simulink model "doc_evm"  (R2014a)
settings: Solver=FixedStepDiscrete  StartTime=0.0  StopTime=(paramEVM.numBursts)*paramEVM.burstLen2*paramEVM.Tnormal  FixedStep=paramEVM.Tnormal  MaxStep=paramEVM.Tnormal  RelTol=1e-3
PreLoadFcn:
  |  paramEVM = doc_evm_init;
undefined symbols (not defined in the file or in its folder): commblksprivate, dfilt, Info
libraries: commrflib2 x3, dsparch4 x2, commutil2 x1, commdigbbndpm3 x1, dspstat3 x1, commrandsrc2 x1, dspsigops x1
CloseFcn:
  | clear paramEVM;
settings Model: Creator=The MathWorks Inc.
settings DataIOCC: SignalLoggingSaveFormat=ModelDataLogs
settings OptimizationCC: ExpressionDepthLimit=2147483647
settings DebuggingCC: UnderspecifiedInitializationDetection=Classic  FcnCallInpInsideContextMsg=UseLocalSettings  StateNameClashWarn=warning  StrictBusMsg=Warning
settings SFSimCC: SimParseCustomCode=off
settings GRTTargetCC: CombineOutputUpdateFcns=off  GRTInterface=on

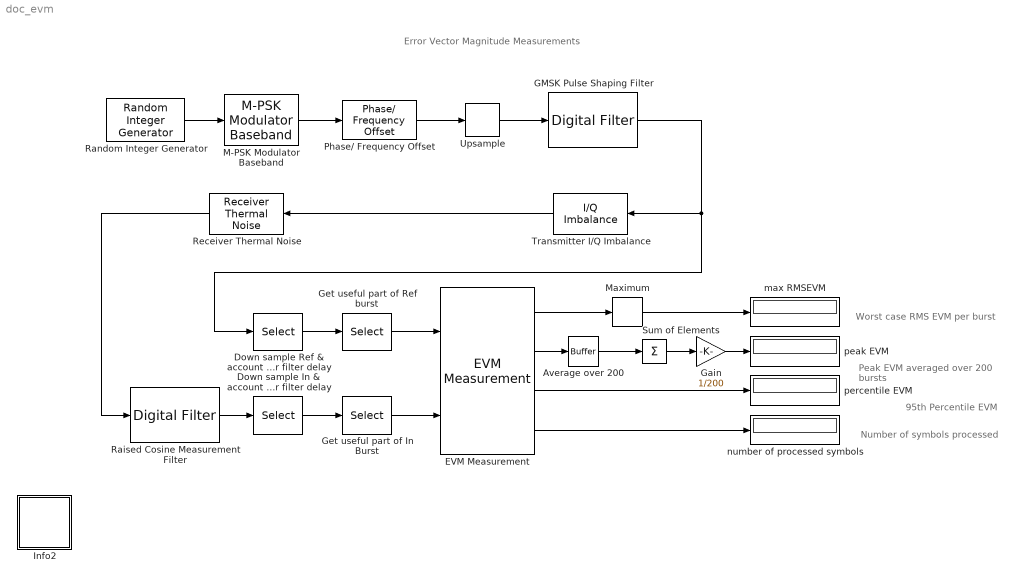
== system doc_evm ==
  note: Error Vector Magnitude Measurements
  note: Worst case
      | RMS EVM per burst
  note: Peak EVM
      | averaged over 200 bursts
  note: 95th Percentile EVM
  note: Number of
      | symbols processed
  Average over 200 : Buffer  N=200  TreatMby1Signals=One channel
  Down sample In & account for filter delay : Selector  NumberOfDimensions=2  InputPortWidth=3  IndexOptions=Index vector (dialog),Select all  Indices=[paramEVM.rcvSigDelay+1:paramEVM.Nsamp:paramEVM.burstLen2*paramEVM.Nsamp],1  OutputSizes=1,1
  Down sample Ref & account for filter delay : Selector  NumberOfDimensions=2  InputPortWidth=3  IndexOptions=Index vector (dialog),Select all  Indices=[paramEVM.refSigDelay+1:paramEVM.Nsamp:paramEVM.burstLen2*paramEVM.Nsamp],1  OutputSizes=1,1
  EVM Measurement : commutil2/EVM Measurement  normMethod=Average reference signal power  averagePower=1  peakPower=1  maxOrMinOut=on  percentileOut=on  percentileVal=95  nSym=on
  GMSK Pulse Shaping Filter : dsparch4/Digital Filter  TypePopup=FIR (all zeros)  IIRFiltStruct=Direct form II transposed  AllPoleFiltStruct=Direct form  FIRFiltStruct=Direct form  CoeffSource=Specify via dialog  NumCoeffs=paramEVM.c0  DenCoeffs=[1 0.1]  BiQuadCoeffs=[1 0.3 0.4 1 0.1 0.2]  LatticeCoeffs=[0.2 0.4]  denIgnore=on  FiltPerSampPopup=One filter per frame  IC=0  ICnum=0  ICden=0  roundingMode=Floor  overflowMode=off  ScaleValues=1  scaleValueFracLength=14  stageInFracLength=15  stageOutFracLength=15  FilterSource=Specify via dialog  dfiltObjectName=dfilt.dffir([1 2 1])  InputProcessing=Columns as channels (frame based)
  Gain : Gain  Gain=1/200
  Get useful part of In Burst : Selector  NumberOfDimensions=2  InputPortWidth=3  IndexOptions=Index vector (dialog),Select all  Indices=[1:paramEVM.burstLen1],1  OutputSizes=1,1
  Get useful part of Ref burst : Selector  NumberOfDimensions=2  InputPortWidth=3  IndexOptions=Index vector (dialog),Select all  Indices=[1:paramEVM.burstLen1],1  OutputSizes=1,1
  Info2 : Subsystem  AncestorBlock=commblksprivate/Info  mask(Info){}
      settings: OpenFcn=helpview([docroot '/toolbox/comm/comm.map'], 'doc_evm')
      mask Display: disp('Info')
  M-PSK Modulator Baseband : commdigbbndpm3/M-PSK Modulator Baseband  M=8  InType=Integer  Enc=User-defined  Mapping=[7 3 2 0 1 5 4 6]  Ph=0  outDtype=double  outWordLen=16  outUDDataType=sfix(16)  outFracLenMode=Best precision  outFracLen=15
  Maximum : dspstat3/Maximum  fcn=Running  reset=None  InputProcessing=Columns as channels (frame based)  indexBase=One  operateOver=Each column  Dimension=1  colComp=on  operation=maximum  roiEnable=off  roiType=Rectangles  roiPortion=Entire ROI  roiOutput=Individual statistics for each ROI  roiFlag=off  accumDataTypeStr=Inherit: Same as product output  accumLastDataTypeStr=Inherit: Same as product output  roundingMode=Floor  overflowMode=off
  Phase/ Frequency Offset : commrflib2/Phase// Frequency Offset  phaseOffset=(0:paramEVM.burstLen2-1)'*paramEVM.phi  freqPort=off  freqOffset=0
  Raised Cosine Measurement Filter : dsparch4/Digital Filter  TypePopup=FIR (all zeros)  IIRFiltStruct=Direct form II transposed  AllPoleFiltStruct=Direct form  FIRFiltStruct=Direct form  CoeffSource=Specify via dialog  NumCoeffs=paramEVM.c1  DenCoeffs=[1 0.1]  BiQuadCoeffs=[1 0.3 0.4 1 0.1 0.2]  LatticeCoeffs=[0.2 0.4]  denIgnore=on  FiltPerSampPopup=One filter per frame  IC=0  ICnum=0  ICden=0  roundingMode=Floor  overflowMode=off  ScaleValues=1  scaleValueFracLength=14  stageInFracLength=15  stageOutFracLength=15  FilterSource=Specify via dialog  dfiltObjectName=dfilt.dffir([1 2 1])  InputProcessing=Columns as channels (frame based)
  Random Integer Generator : commrandsrc2/Random Integer Generator  mul=8  seed=37  Ts=paramEVM.Tnormal  frameBased=on  sampPerFrame=paramEVM.burstLen2  orient=off  outDataType=double
  Receiver Thermal Noise : commrflib2/Receiver Thermal Noise  method=Noise temperature  ntemp=290  nfigure=3.01  nfactor=2  seed=67987
  Sum of Elements : Sum  Inputs=+  CollapseMode=Specified dimension
  Transmitter I/Q Imbalance : commrflib2/I//Q Imbalance  ampImbal=0.5  phsImbal=1  Idc=0  Qdc=0
  Upsample : dspsigops/Upsample  N=paramEVM.Nsamp  phase=0  InputProcessing=Columns as channels (frame based)  RateOptions=Enforce single-rate processing  ic=0  mode=Unused parameter value
  max RMSEVM : Display
  number of processed symbols : Display
  peak EVM : Display
  percentile EVM : Display
  wires:
  Random Integer Generator/1 -> M-PSK Modulator Baseband/1
  M-PSK Modulator Baseband/1 -> Phase/ Frequency Offset/1
  Upsample/1 -> GMSK Pulse Shaping Filter/1
  Phase/ Frequency Offset/1 -> Upsample/1
  Average over 200/1 -> Sum of Elements/1
  Sum of Elements/1 -> Gain/1
  Gain/1 -> peak EVM/1
  EVM Measurement/3 -> percentile EVM/1
  EVM Measurement/4 -> number of processed symbols/1
  EVM Measurement/2 -> Average over 200/1
  GMSK Pulse Shaping Filter/1 -> Transmitter I/Q Imbalance/1, Down sample Ref & account for filter delay/1
  Transmitter I/Q Imbalance/1 -> Receiver Thermal Noise/1
  Raised Cosine Measurement Filter/1 -> Down sample In & account for filter delay/1
  Down sample In & account for filter delay/1 -> Get useful part of In Burst/1
  Get useful part of In Burst/1 -> EVM Measurement/2
  Receiver Thermal Noise/1 -> Raised Cosine Measurement Filter/1
  Down sample Ref & account for filter delay/1 -> Get useful part of Ref burst/1
  Get useful part of Ref burst/1 -> EVM Measurement/1
  EVM Measurement/1 -> Maximum/1
  Maximum/1 -> max RMSEVM/1

== system doc_evm/Info2 ==
